simulink model "sos_3"  (Simulink 6.1)
settings: Solver=ode45  StartTime=0.0  StopTime=10.0  RelTol=1e-3
libraries: dspsigops x2
settings Model: Creator=svenhoffmann  LastModifiedBy=svenhoffmann  ExtModeAutoUpdateStatusClock=off
settings DebuggingCC: SolverPrmCheckMsg=warning

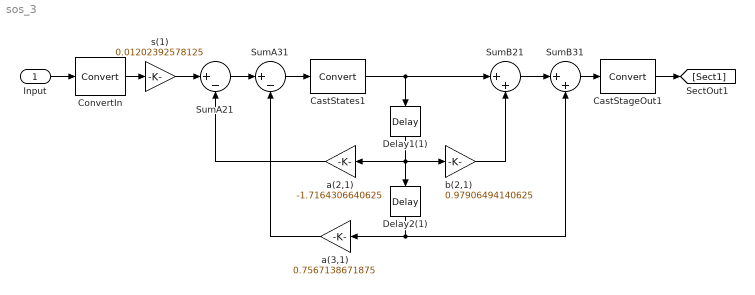
== system sos_3 ==
  Input : Inport  Port=1  LatchInput=off
  CastStageOut1 : DataTypeConversion  OutDataTypeMode=Specify via dialog  OutScaling=2^-11  RndMeth=Nearest  LockScale=on
  CastStates1 : DataTypeConversion  OutDataTypeMode=Specify via dialog  OutScaling=2^-15  RndMeth=Nearest  LockScale=on
  ConvertIn : DataTypeConversion  OutDataTypeMode=Specify via dialog  OutScaling=2^-15  RndMeth=Nearest  SaturateOnIntegerOverflow=on  LockScale=on
  Delay1(1) : dspsigops/Delay  Orientation=down  dly_unit=Samples  delay=1  ic_detail=off  dif_ic_for_ch=off  dif_ic_for_dly=off  ic=0  reset_popup=None
  Delay2(1) : dspsigops/Delay  Orientation=down  dly_unit=Samples  delay=1  ic_detail=off  dif_ic_for_ch=off  dif_ic_for_dly=off  ic=0  reset_popup=None
  SumA21 : Sum  Inputs=|+-  OutDataTypeMode=Specify via dialog  OutDataType=sfix(40)  OutScaling=2^-29  RndMeth=Nearest  LockScale=on
  SumA31 : Sum  Inputs=|+-  OutDataTypeMode=Specify via dialog  OutDataType=sfix(40)  OutScaling=2^-29  RndMeth=Nearest  LockScale=on
  SumB21 : Sum  Inputs=|++  OutDataTypeMode=Specify via dialog  OutDataType=sfix(40)  OutScaling=2^-29  RndMeth=Nearest  LockScale=on
  SumB31 : Sum  Inputs=|++  OutDataTypeMode=Specify via dialog  OutDataType=sfix(40)  OutScaling=2^-29  RndMeth=Nearest  LockScale=on
  a(2,1) : Gain  Orientation=left  Gain=-1.7164306640625  ParameterDataTypeMode=Specify via dialog  ParameterScalingMode=Use specified scaling  ParameterScaling=2^-14  OutDataTypeMode=Specify via dialog  OutDataType=sfix(32)  OutScaling=2^-29  RndMeth=Nearest  LockScale=on
  a(3,1) : Gain  Orientation=left  Gain=0.7567138671875  ParameterDataTypeMode=Specify via dialog  ParameterScalingMode=Use specified scaling  ParameterScaling=2^-14  OutDataTypeMode=Specify via dialog  OutDataType=sfix(32)  OutScaling=2^-29  RndMeth=Nearest  LockScale=on
  b(2,1) : Gain  Gain=0.97906494140625  ParameterDataTypeMode=Specify via dialog  ParameterScalingMode=Use specified scaling  ParameterScaling=2^-14  OutDataTypeMode=Specify via dialog  OutDataType=sfix(32)  OutScaling=2^-29  RndMeth=Nearest  LockScale=on
  s(1) : Gain  Gain=0.01202392578125  ParameterDataTypeMode=Specify via dialog  ParameterScalingMode=Use specified scaling  ParameterScaling=2^-14  OutDataTypeMode=Specify via dialog  OutScaling=2^-9  RndMeth=Nearest  LockScale=on
  wires:
  Input/1 -> ConvertIn/1
  ConvertIn/1 -> s(1)/1
  s(1)/1 -> SumA21/1
  SumA21/1 -> SumA31/1
  SumA31/1 -> CastStates1/1
  CastStates1/1 -> SumB21/1, Delay1(1)/1
  SumB21/1 -> SumB31/1
  CastStageOut1/1 -> [Sect1]
  SumB31/1 -> CastStageOut1/1
  Delay1(1)/1 -> a(2,1)/1, b(2,1)/1, Delay2(1)/1
  b(2,1)/1 -> SumB21/2
  Delay2(1)/1 -> SumB31/2, a(3,1)/1
  a(2,1)/1 -> SumA21/2
  a(3,1)/1 -> SumA31/2
